simulink model "PMSM_My_PI_Simscapes"  (R2017b)
settings: Solver=VariableStepAuto  StartTime=0.0  StopTime=0.2  FixedStep=0.000001  MaxStep=1e-4  RelTol=1e-3
undefined symbols (not defined in the file or in its folder): sigbuilder_block
libraries: fl_lib x46, nesl_utility x28, elec_lib x13, powerlib x2, simulink x1
settings Model: Creator=Linyc  LastModifiedBy=Crazyyiwen
settings DebuggingCC: UnconnectedLineMsg=none

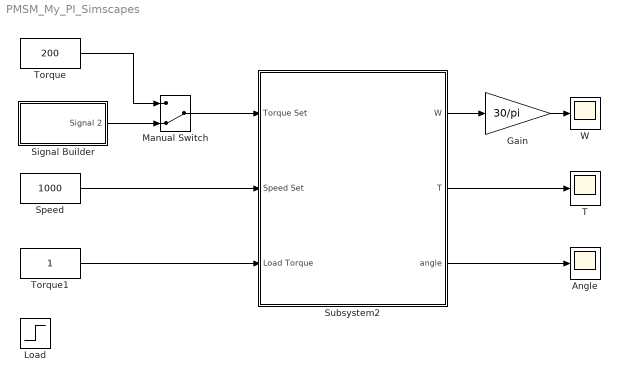
== system PMSM_My_PI_Simscapes ==
  Angle : Scope
  Gain : Gain  Gain=30/pi
  Load : Step  Time=0.02  After=0  SampleTime=0
  Manual Switch : ManualSwitch  CurrentSetting=0
  Signal Builder : Subsystem  Tag=STV Subsys  LoadFcn=sigbuilder_block('load');  StartFcn=sigbuilder_block('start');  StopFcn=sigbuilder_block('stop');  ClipboardFcn=sigbuilder_block('clipboard');  mask(Sigbuilder block){tuvar=[0:10]}
      mask help: Simulink:masks:SigbuilderBlock_MD
      mask init:
      | if ~strcmp(get_param(bdroot(gcbh),'SimulationStatus'),'stopped') tuvar = sigbuilder_block('maskInit'); end
      settings: CopyFcn=sigbuilder_block('copy');  DeleteFcn=sigbuilder_block('delete');  ModelCloseFcn=sigbuilder_block('modelClose');  PreSaveFcn=sigbuilder_block('preSave');  PauseFcn=sigbuilder_block('pause');  ContinueFcn=sigbuilder_block('continue');  NameChangeFcn=sigbuilder_block('namechange');  OpenFcn=sigbuilder_block('open',[424.5 166.5 847.5 399.75 ]);  CloseFcn=sigbuilder_block('close');
      mask Display: plot(0, 0, 100, 100,[2, 2, 32, 32, 2], [68, 8, 8, 68, 68],[32, 2], [38, 38], [32, 19, 2],[53, 60, 44], [32, 17, 17, 2],[16, 16, 31, 31]);txt = getActiveGroup(gcbh);text(2, 100, txt,'verticalAlignment', 'top');
  Speed : Constant  Value=1000
  Subsystem2 : Subsystem
  T : Scope
  Torque : Constant  Value=200
  Torque1 : Constant
  W : Scope
  wires:
  Speed/1 -> Subsystem2/2(Speed Set)
  Subsystem2/1(W) -> Gain/1
  Subsystem2/2(T) -> T/1
  Subsystem2/3(angle) -> Angle/1
  Gain/1 -> W/1
  Torque/1 -> Manual Switch/1
  Manual Switch/1 -> Subsystem2/1(Torque Set)
  Signal Builder/1(Signal 2) -> Manual Switch/2
  Torque1/1 -> Subsystem2/3(Load Torque)

== system PMSM_My_PI_Simscapes/Signal Builder ==
  Demux : Demux  Tag=STV Demux  Outputs=1
  FromWs : FromWorkspace  Tag=STV FromWs  VariableName=tuvar  SampleTime=0
      SigBuilderData=|
      | common.afterFinalStr = 'Extrapolate'
      | common.sampleTime = 0
      | dataSet.timeRange = [0 2]
      | dataSet.name = 'Group 1'
      | sbobj.Groups.Name = 'Group 1'
      | sbobj.Groups.Signals.Name = 'Signal 2'
      | sbobj.Groups.Signals.XData = [0 1 1 2]
      | sbobj.Groups.Signals.YData = [200 200 0 0]
      | sbobj.Groups.TimeRange = [0 2]
  Signal 2 : Outport  Tag=STV Outport
  wires:
  FromWs/1 -> Demux/1
  Demux/1 -> Signal 2/1

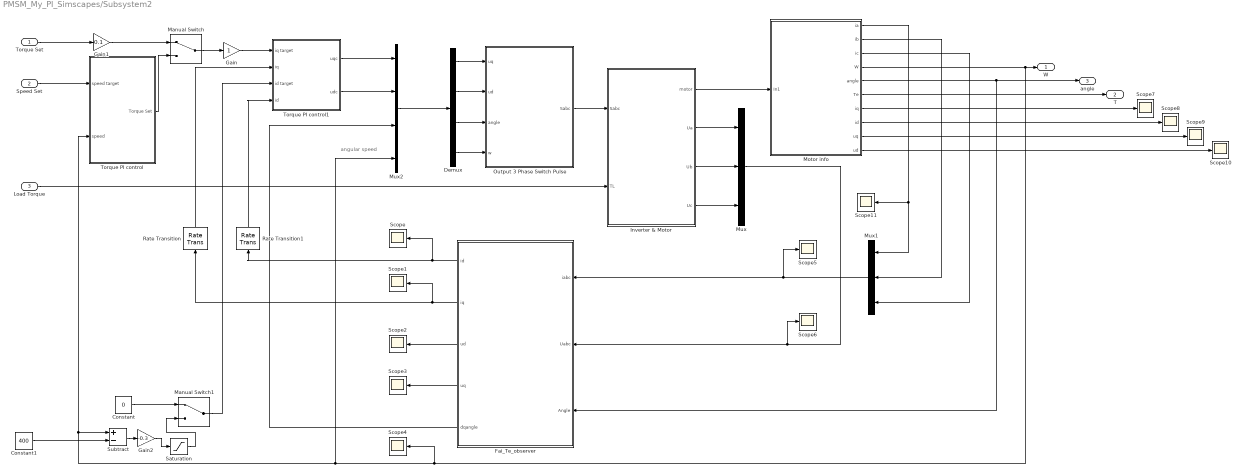
== system PMSM_My_PI_Simscapes/Subsystem2 ==
  note: angular speed
  Torque Set : Inport
  Speed Set : Inport  Port=2
  Load Torque : Inport  Port=3
  Constant : Constant  Value=0
  Constant1 : Constant  Value=400
  Demux : Demux
  Fai_Te_observer : Subsystem
  Gain : Gain
  Gain1 : Gain  Gain=0.1
  Gain2 : Gain  Gain=-0.3
  Inverter & Motor : Subsystem
  Manual Switch : ManualSwitch
  Manual Switch1 : ManualSwitch
  Motor info : Subsystem
  Mux : Mux  Inputs=3
  Mux1 : Mux  Inputs=3
  Mux2 : Mux
  Output 3 Phase Switch Pulse : Subsystem
  Rate Transition : RateTransition  OutPortSampleTime=0.0002
  Rate Transition1 : RateTransition  OutPortSampleTime=0.0002
  Saturation : Saturate  UpperLimit=0  LowerLimit=-150
  Scope{,1..11} (12 alike) : Scope
  Subtract : Sum  Inputs=+-
  Torque PI control : Subsystem
  Torque PI control1 : Subsystem
  W : Outport
  T : Outport  Port=2
  angle : Outport  Port=3
  wires:
  Motor info/4(W) -> Scope4/1, Mux2/4, Subtract/1, Torque PI control/2(speed), W/1
  Load Torque/1 -> Inverter & Motor/2(TL)
  Inverter & Motor/2(Ua) -> Mux/1
  Inverter & Motor/4(Uc) -> Mux/3
  Inverter & Motor/3(Ub) -> Mux/2
  Motor info/6(Te) -> T/1
  Inverter & Motor/1(motor) -> Motor info/1(In1)
  Motor info/5(angle) -> Fai_Te_observer/3(Angle), angle/1
  Motor info/1(ia) -> Scope11/1, Mux1/1
  Motor info/2(ib) -> Mux1/2
  Motor info/3(ic) -> Mux1/3
  Output 3 Phase Switch Pulse/1(Sabc) -> Inverter & Motor/1(Sabc)
  Mux1/1 -> Fai_Te_observer/1(iabc), Scope5/1
  Mux/1 -> Fai_Te_observer/2(Uabc), Scope6/1
  Mux2/1 -> Demux/1
  Motor info/7(iq) -> Scope7/1
  Motor info/8(id) -> Scope8/1
  Motor info/9(uq) -> Scope9/1
  Motor info/10(ud) -> Scope10/1
  Fai_Te_observer/1(id) -> Rate Transition1/1, Scope/1
  Fai_Te_observer/2(iq) -> Rate Transition/1, Scope1/1
  Fai_Te_observer/3(ud) -> Scope2/1
  Fai_Te_observer/4(uq) -> Scope3/1
  Speed Set/1 -> Torque PI control/1(speed target)
  Torque Set/1 -> Gain1/1
  Torque PI control/1(Torque Set) -> Manual Switch/2
  Fai_Te_observer/5(dqangle) -> Mux2/3
  Manual Switch/1 -> Gain/1
  Gain/1 -> Torque PI control1/1(iq target)
  Demux/1 -> Output 3 Phase Switch Pulse/1(uq)
  Demux/2 -> Output 3 Phase Switch Pulse/2(ud)
  Demux/3 -> Output 3 Phase Switch Pulse/3(angle)
  Torque PI control1/1(uqc) -> Mux2/1
  Rate Transition/1 -> Torque PI control1/2(iq)
  Demux/4 -> Output 3 Phase Switch Pulse/4(w)
  Gain1/1 -> Manual Switch/1
  Torque PI control1/2(udc) -> Mux2/2
  Rate Transition1/1 -> Torque PI control1/4(id)
  Constant/1 -> Manual Switch1/1
  Manual Switch1/1 -> Torque PI control1/3(id target)
  Constant1/1 -> Subtract/2
  Subtract/1 -> Gain2/1
  Gain2/1 -> Saturation/1
  Saturation/1 -> Manual Switch1/2

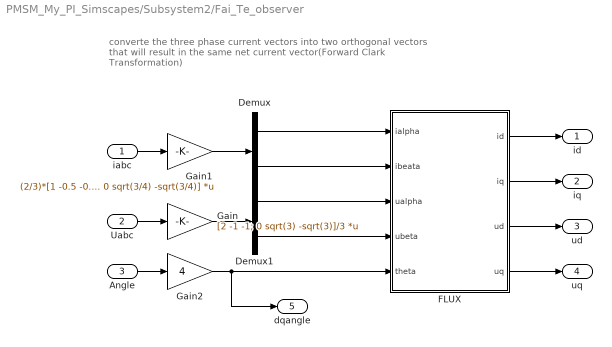
== system PMSM_My_PI_Simscapes/Subsystem2/Fai_Te_observer ==
  note: converte the three phase current vectors into
      | two orthogonal vectors that will result in the
      | same net current vector(Forward Clark Transformation)
  iabc : Inport
  Uabc : Inport  Port=2
  Angle : Inport  Port=3
  Demux : Demux  Outputs=2
  Demux1 : Demux  Outputs=2
  FLUX : Subsystem
  Gain : Gain  Gain=[2 -1 -1; 0 sqrt(3) -sqrt(3)]/3  Multiplication=Matrix(K*u)
  Gain1 : Gain  Gain=(2/3)*[1 -0.5 -0.5; 0 sqrt(3/4) -sqrt(3/4)]  Multiplication=Matrix(K*u)
  Gain2 : Gain  Gain=4
  id : Outport
  iq : Outport  Port=2
  ud : Outport  Port=3
  uq : Outport  Port=4
  dqangle : Outport  Port=5
  wires:
  Demux/1 -> FLUX/1(ialpha)
  Gain/1 -> Demux1/1
  iabc/1 -> Gain1/1
  Demux/2 -> FLUX/2(ibeata)
  Demux1/2 -> FLUX/4(ubeta)
  Demux1/1 -> FLUX/3(ualpha)
  Uabc/1 -> Gain/1
  Gain1/1 -> Demux/1
  Angle/1 -> Gain2/1
  Gain2/1 -> dqangle/1, FLUX/5(theta)
  FLUX/1(id) -> id/1
  FLUX/2(iq) -> iq/1
  FLUX/3(ud) -> ud/1
  FLUX/4(uq) -> uq/1

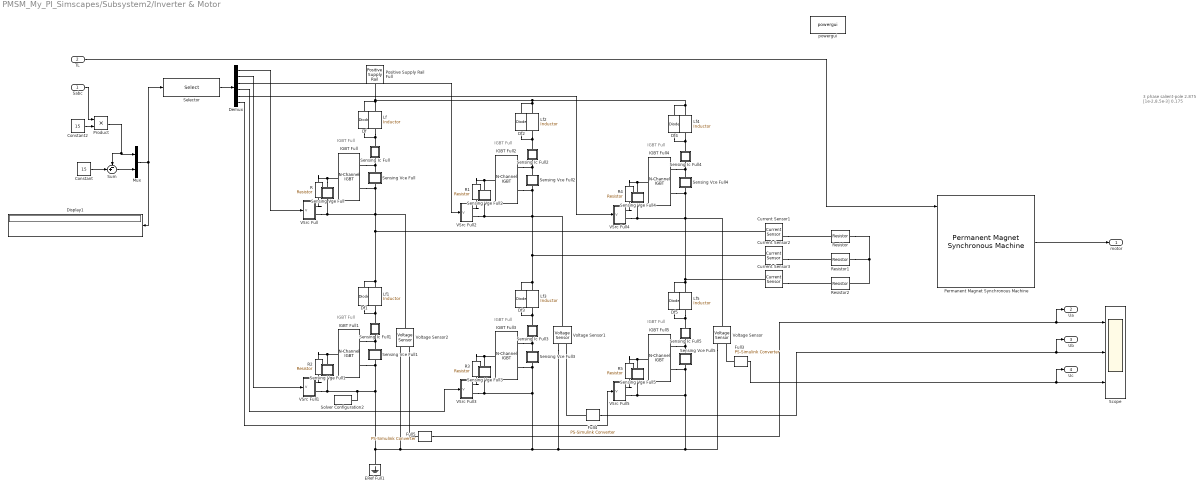
== system PMSM_My_PI_Simscapes/Subsystem2/Inverter & Motor ==
  note: 3 phase
      | salient-pole
      |
      | 2.875
      | [1e-2,8.5e-3]
      | 0.175
  note: IGBT
      | Full
  note: IGBT
      | Full
  note: IGBT
      | Full
  note: IGBT
      | Full
  note: IGBT
      | Full
  note: IGBT
      | Full
  Sabc : Inport
  TL : Inport  Port=2
  Constant : Constant  Value=15
  Constant2 : Constant  Value=15
  Current Sensor1 : fl_lib/Electrical/Electrical Sensors/Current Sensor
      settings: SourceProductName=Foundation Library
  Current Sensor2 : fl_lib/Electrical/Electrical Sensors/Current Sensor
      settings: SourceProductName=Foundation Library
  Current Sensor3 : fl_lib/Electrical/Electrical Sensors/Current Sensor
      settings: SourceProductName=Foundation Library
  Demux : Demux  Outputs=6
  Df{,1..5} (6 alike) : elec_lib/Semiconductor Devices/Diode  ModelType=3  Vf=0.6 V  Ron=0.01 Ohm  Goff=1e-5 S  Rz=0.3 Ohm  Vz=50 V  C_PWL=50 pF  prmExp=1  I12="[ 3  30 ] A"  V12=[ 0.8 1.1 ] V  I1=0.0137 A  V1=0.6 V  IS=1e-12 A  ec=1  RS=0.01 Ohm  Tmeas=25 degC  BV=Inf V  C_param=1  CJ0=1 nF  VJ=1 V  Mgrad=0.5  Vvec=[ 0.1 10 100 ] V  Cvec=[ 3.5 1 0.4 ] pF  FC=0.5  Q_param=2  Irrm=-100 A  iF=200 A  didt=-1000 A/us  trr=115 ns  TT=50 ns  tau=100 ns  T_param=1  IS_T2=1.25e-7 A  I1_T2=0.245 A  V1_T2=0.5 V  Tmeas2=125 degC  EG_param=1  EG=1.11 eV  XTI_param=1  XTI=3  dBVdT=0 V/K  Tdevice=25 degC  i_capacitor_specify=off  i_capacitor_priority=High  i_capacitor=0 A  i_capacitor_nominal_specify=off  i_capacitor_nominal_unit=A  i_capacitor_nominal_value=1  v_capacitor_specify=off  v_capacitor_priority=None  v_capacitor=0 V  v_capacitor_nominal_specify=off  v_capacitor_nominal_unit=V  v_capacitor_nominal_value=1  Rth=[ 0 10 ] K/W  thermal_mass_parameterization=1  thermal_mass=[ 0 1 ] J/K  thermal_time_constant=[ 0 10 ] s  thermal_mass_initial_temperatures=[ 25 25 ] degC
      settings: SourceProductName=Simscape Electronics  SourceProductBaseCode=SN
  Display1 : Display
  ERef Full1 : fl_lib/Electrical/Electrical Elements/Electrical Reference
      settings: SourceProductName=Foundation Library
  Full3 : nesl_utility/PS-Simulink Converter  PhysicalDomain=network_engine_domain  SubClassName=ps_output  LeftPortType=input  RightPortType=output  PseudoPeriodic=off  Frequencies=[]  Unit=1  AffineConversion=off
  Full4 : nesl_utility/PS-Simulink Converter  PhysicalDomain=network_engine_domain  SubClassName=ps_output  LeftPortType=input  RightPortType=output  PseudoPeriodic=off  Frequencies=[]  Unit=1  AffineConversion=off
  Full5 : nesl_utility/PS-Simulink Converter  PhysicalDomain=network_engine_domain  SubClassName=ps_output  LeftPortType=input  RightPortType=output  PseudoPeriodic=off  Frequencies=[]  Unit=1  AffineConversion=off
  IGBT Full{,1..5} (6 alike) : elec_lib/Semiconductor Devices/N-Channel IGBT  model_type=1  Ices=2 mA  Vces=600 V  Vth=6 V  Vce_sat=2.6 V  Ice_sat=300 A  Vge_sat=15 V  ec=3  Tmeas=25 degC  Vge_vec=[ -2 6 7 8 10 12 15 20 ] V  Vce_vec=[0, 1.1, 1.3, 1.45, 1.75, 2.25, 2.7] V  T_vec=[25, 125] degC  Ic_mat=[ -1.015e-5 1.35e-8 4.7135e-4 5.092e-4 5.105e-4 5.117500000000001e-4 5.1299e-4 5.1423e-4 5.1548e-4 5.1672e-4; -9.986899999999999e-6 1.35e-8 4.7135e-4 5.092e-4 5.105e-4 5.117500000000001e-4 5.1299e-4 5.1423e-4 5.1548e-4 5.1672e-4; -9.955e-6 1.35e-8 0.0065225 3.3324 48.154 93.661 105.52 105.72 105.93 106.14; -9.955e-6 1.35e-8 0.0065235 3.5783 70.264 166.33 252.4 317.67 353.38 357.39; -9.955e-6 1.35e-8 0.006524 3.7206 89.17100000000001 228.09 371.63 511.02 642.6900000000001 764.04; -9.9549e-6 1.35e-8 0.0065242 3.7716 97.79300000000001 256.21 424.27 592.92 759.2 921.52; -9.9549e-6 1.35e-8 0.0065243 3.8067 104.52 278.11 464.6 654.37 844.5700000000001 1.0339e+3; -9.9549e-6 1.35e-8 0.0065244 3.8324 109.92 295.67 496.54 702.28 909.96 1.1183e+3 ] A  Ic_mat_3D=zeros(8, 10, 2) A  C_param=1  C_GE=23.7 nF  C_GC=2.7 nF  C_CE=0 nF  C_ies=26.4 nF  C_res=2.7 nF  C_oes=0 nF  C_GE_vec=[ 25 31 26.5 24.9 25 24.9 24.6 24.7 24.8 ] nF  C_GC_vec=[ 55 9 5.5 3.1 2.5 2.1 1.9 1.8 1.7 ] nF  C_CE_vec=[ 5 11 6.5 4.9 3.5 2.7 2.1 1.7 1.4 ] nF  C_ies_vec=[ 80 40 32 28 27.5 27 26.5 26.5 26.5 ] nF  C_res_vec=[ 55 9 5.5 3.1 2.5 2.1 1.9 1.8 1.7 ] nF  C_oes_vec=[ 55 20 12 8 6 4.8 4 3.5 3.1 ] nF  C_Vce_vec=[ 0 1 2 5 10 15 20 25 30 ] V  charge_linearity_param=2  C_OX=50 nF  V_C_OX=-4 V  TF=150 us  VAF=200 V  RC=0.001 Ohm  RE=0.001 Ohm  RG=0.001 Ohm  BF=1  T_param=1  Ices_T2=100 mA  EG=1.11 eV  Vce_sat_T2=3 V  Tmeas2=125 degC  XTI=3  BEX=-1.5  RG_alpha=0 1/K  Tdevice=25 degC  Tdevice_3D=25 degC  Rth=[0, 10] K/W  thermal_mass_parameterization=1  thermal_mass=[0, 1] J/K  thermal_time_constant=[0, 10] s  thermal_mass_initial_temperatures=[298.15, 298.15] K  Ic_vec1=[0, 10, 50, 100, 200, 400, 600] A  Vce_vec1=[0, 1.1, 1.3, 1.45, 1.75, 2.25, 2.7] V  Rmiller=0.12 Ohm  Goff=1e-5 1/Ohm  t_on=0.09 us  t_rise=0.7 us  t_off=0.2 us  t_fall=0.4 us  v_meas=300 V  Tj_vec1=[298.15, 398.15] K  Vce_mat1=[0, 1.1, 1.3, 1.45, 1.75, 2.25, 2.7; 0, 1.0, 1.15, 1.35, 1.7, 2.35, 3.0] V  E_turn_on_mat1=[0, 0.2, 1, 2, 4, 8, 15; 0, 0.3, 1.3, 2.5, 5, 11, 18] * 1e-3 J  E_turn_off_mat1=[0, 0.3, 1.5, 3, 6, 15, 25; 0, 0.7, 3.3, 6.5, 13, 25, 35] * 1e-3 J
      settings: SourceProductName=Simscape Electronics  SourceProductBaseCode=SN
  Lf{,1..5} (6 alike) : fl_lib/Electrical/Electrical Elements/Inductor  l=0.5e-5 H  r=1e-4 Ohm  g=1e-6 1/Ohm  i_specify=off  i_priority=High  i=0 A  i_nominal_specify=off  i_nominal_unit=A  i_nominal_value=1  v_specify=off  v_priority=High  v=0 V  v_nominal_specify=off  v_nominal_unit=V  v_nominal_value=1  i_L_specify=on  i_L_priority=High  i_L=0 A  i_L_nominal_specify=off  i_L_nominal_unit=A  i_L_nominal_value=1
      settings: SourceProductName=Foundation Library
  Mux : Mux  Inputs=2
  Permanent Magnet Synchronous Machine : powerlib/Machines/Permanent Magnet Synchronous Machine  NbPhases=3  FluxDistribution=Sinusoidal  RotorType=Salient-pole  MechanicalLoad=Torque Tm  PresetModel=No  ShowDetailedParameters=on  MeasurementBus=off  Resistance=2.875  Inductance=8.5e-3  dqInductances=[1e-2,8.5e-3]  La=0.000395  MachineConstant=Flux linkage established by magnets (V.s)  Flux=0.175  VoltageCst=126.966  TorqueCst=1.05  Flat=120  Mechanical=[0.0027 0.175 4 0]  PolePairs=2  InitialConditions=[0,0, 0,0]  InitialConditions5ph=[0 0 0 0 0 0]  TsPowergui=0  TsBlock=-1  RefAngle=Aligned with phase A axis (original Park)
      settings: SourceProductName=Simscape Power Systems
  Positive Supply Rail Full : elec_lib/Sources/Positive Supply Rail  v0=380 V
      settings: SourceProductName=Simscape Electronics  SourceProductBaseCode=SN
  Product : Product
  R{,1..5} (6 alike) : fl_lib/Electrical/Electrical Elements/Resistor  R=4.7 Ohm  i_specify=off  i_priority=High  i=0 A  i_nominal_specify=off  i_nominal_unit=A  i_nominal_value=1  v_specify=off  v_priority=High  v=0 V  v_nominal_specify=off  v_nominal_unit=V  v_nominal_value=1
      settings: SourceProductName=Foundation Library
  Resistor : fl_lib/Electrical/Electrical Elements/Resistor  R=5 Ohm  i_specify=off  i_priority=None  i=0 A  i_nominal_specify=off  i_nominal_unit=A  i_nominal_value=1  v_specify=off  v_priority=None  v=0 V  v_nominal_specify=off  v_nominal_unit=V  v_nominal_value=1
  Resistor1 : fl_lib/Electrical/Electrical Elements/Resistor  R=5 Ohm  i_specify=off  i_priority=None  i=0 A  i_nominal_specify=off  i_nominal_unit=A  i_nominal_value=1  v_specify=off  v_priority=None  v=0 V  v_nominal_specify=off  v_nominal_unit=V  v_nominal_value=1
  Resistor2 : fl_lib/Electrical/Electrical Elements/Resistor  R=5 Ohm  i_specify=off  i_priority=None  i=0 A  i_nominal_specify=off  i_nominal_unit=A  i_nominal_value=1  v_specify=off  v_priority=None  v=0 V  v_nominal_specify=off  v_nominal_unit=V  v_nominal_value=1
  Scope : Scope  NumInputPorts=3
  Selector : Selector  InputPortWidth=6  IndexOptions=Index vector (dialog)  Indices=[1 4 2 5 3 6]  OutputSizes=1
  Sensing Ic Full : Subsystem
      mask Display: disp('Ic')
  Sensing Ic Full1 : Subsystem
      mask Display: disp('Ic')
  Sensing Ic Full2 : Subsystem
      mask Display: disp('Ic')
  Sensing Ic Full3 : Subsystem
      mask Display: disp('Ic')
  Sensing Ic Full4 : Subsystem
      mask Display: disp('Ic')
  Sensing Ic Full5 : Subsystem
      mask Display: disp('Ic')
  Sensing Vce Full : Subsystem
      mask Display: disp('Vce')
  Sensing Vce Full1 : Subsystem
      mask Display: disp('Vce')
  Sensing Vce Full2 : Subsystem
      mask Display: disp('Vce')
  Sensing Vce Full3 : Subsystem
      mask Display: disp('Vce')
  Sensing Vce Full4 : Subsystem
      mask Display: disp('Vce')
  Sensing Vce Full5 : Subsystem
      mask Display: disp('Vce')
  Sensing Vge Full : Subsystem
      mask Display: disp('Vge')
  Sensing Vge Full1 : Subsystem
      mask Display: disp('Vge')
  Sensing Vge Full2 : Subsystem
      mask Display: disp('Vge')
  Sensing Vge Full3 : Subsystem
      mask Display: disp('Vge')
  Sensing Vge Full4 : Subsystem
      mask Display: disp('Vge')
  Sensing Vge Full5 : Subsystem
      mask Display: disp('Vge')
  Solver Configuration2 : nesl_utility/Solver Configuration  PhysicalDomain=network_engine_domain  SubClassName=solver  LeftPortType=input  RightPortType=generic  Accelerate=off  Tones=[]  Harmonics=[]  SimulateNoise=off  Profile=off  UseLocalSampling=off  EnableSwitchedLinearOptims=on  FrequencyDomain=off  UseCCode=off  RelTol=0.001  AbsTol=1e-06  MinStep=1e-09  ToWorkspace=off  RevertToSquareIcSolve=off  NumHomotopyIterations=100  PhasorMode=off  PhasorModeNumHarmonics=1  DoDC=off  ResidualTolerance=1e-6  UseLocalSolver=off  LocalSolverChoice=NE_BACKWARD_EULER_ADVANCER  LocalSolverSampleTime=1e-6  DoFixedCost=off  MaxNonlinIter=3  MaxModeIter=2  LinearAlgebra=Sparse  DelaysMemoryBudget=1024  AutomaticFiltering=on  FilteringTimeConstant=0.001
  Sum : Sum  Inputs=-+|
  VSrc Full : Subsystem
      settings: CopyFcn=set_param(gcb,'LinkStatus','none')
  VSrc Full1 : Subsystem
      settings: CopyFcn=set_param(gcb,'LinkStatus','none')
  VSrc Full2 : Subsystem
      settings: CopyFcn=set_param(gcb,'LinkStatus','none')
  VSrc Full3 : Subsystem
      settings: CopyFcn=set_param(gcb,'LinkStatus','none')
  VSrc Full4 : Subsystem
      settings: CopyFcn=set_param(gcb,'LinkStatus','none')
  VSrc Full5 : Subsystem
      settings: CopyFcn=set_param(gcb,'LinkStatus','none')
  Voltage Sensor : fl_lib/Electrical/Electrical Sensors/Voltage Sensor
      settings: SourceProductName=Foundation Library
  Voltage Sensor1 : fl_lib/Electrical/Electrical Sensors/Voltage Sensor
      settings: SourceProductName=Foundation Library
  Voltage Sensor2 : fl_lib/Electrical/Electrical Sensors/Voltage Sensor
      settings: SourceProductName=Foundation Library
  powergui : powerlib/powergui  Priority=1  SimulationMode=Continuous  SampleTime=0.000001  frequency=60  Iterations=50  frequencyindice=0  Pbase=100e6  ErrMax=1e-4  UnitsV=kV  UnitsW=MW  buscounter=0  FunctionMessages=off  echomessages=off  EnableUseOfTLC=off  CurrentSourceSwitches=off  DisableSnubberDevices=off  DisableRonSwitches=off  DisableVfSwitches=off  DisplayEquations=off  SolverType=Tustin/Backward Euler (TBE)  Interpol=off  ExternalGateDelay=off  methode=off  Ts=100  x0status=blocks  SPID=on  SwTol=0  HookPort=off  RestoreLinks=warning  ResistiveCurrentMeasurement=off  Frange=[0:2:500]  Ylog=off  Xlog=on  ShowGrid=off  save=off  variable=ZData  structure=0  ZoomFFT=off  StartTime=0.0  cycles=1  DisplayStyle=1  fundamental=60  FreqAxis=off  MaxFrequency=1000  frequencyindicesteady=1  RmsSteady=1  display=off
  motor : Outport
  Ua : Outport  Port=2
  Ub : Outport  Port=3
  Uc : Outport  Port=4
  wires:
  Constant/1 -> Sum/2
  Sum/1 -> Mux/2
  Mux/1 -> Display1/1, Selector/1
  Full5/1 -> Ua/1, Scope/1
  Full4/1 -> Ub/1, Scope/2
  Full3/1 -> Uc/1, Scope/3
  Permanent Magnet Synchronous Machine/1 -> motor/1
  Selector/1 -> Demux/1
  Constant2/1 -> Product/2
  Sabc/1 -> Product/1
  Product/1 -> Sum/1, Mux/1
  Demux/1 -> VSrc Full/1(V)
  Demux/2 -> VSrc Full1/1(V)
  Demux/3 -> VSrc Full2/1(V)
  Demux/4 -> VSrc Full3/1(V)
  Demux/5 -> VSrc Full4/1(V)
  Demux/6 -> VSrc Full5/1(V)
  TL/1 -> Permanent Magnet Synchronous Machine/1
  connections:
  Sensing Vge Full/LConn1 -- R/RConn1 -- IGBT Full/LConn1
  Df3/RConn1 -- Current Sensor2/LConn1 -- Sensing Vge Full2/RConn1 -- VSrc Full2/RConn2 -- Voltage Sensor1/LConn1 -- Sensing Vce Full2/RConn1 -- IGBT Full2/RConn2 -- Lf3/LConn1
  Sensing Vce Full5/LConn1 -- IGBT Full5/RConn1 -- Sensing Ic Full5/RConn1
  IGBT Full2/LConn1 -- Sensing Vge Full2/LConn1 -- R1/RConn1
  Lf4/RConn1 -- Sensing Ic Full4/LConn1 -- Df4/LConn1
  Lf2/RConn1 -- Sensing Ic Full2/LConn1 -- Df2/LConn1
  Lf1/RConn1 -- Sensing Ic Full1/LConn1 -- Df1/LConn1
  R3/RConn1 -- IGBT Full3/LConn1 -- Sensing Vge Full3/LConn1
  Df5/RConn1 -- Current Sensor3/LConn1 -- Sensing Vge Full4/RConn1 -- VSrc Full4/RConn2 -- Voltage Sensor/LConn1 -- Sensing Vce Full4/RConn1 -- IGBT Full4/RConn2 -- Lf5/LConn1
  IGBT Full3/RConn2 -- Voltage Sensor/RConn2 -- Sensing Vge Full5/RConn1 -- VSrc Full5/RConn2 -- Sensing Vce Full5/RConn1 -- IGBT Full5/RConn2 -- Voltage Sensor1/RConn2 -- Voltage Sensor2/RConn2 -- Sensing Vce Full1/RConn1 -- IGBT Full1/RConn2 -- Solver Configuration2/RConn1 -- VSrc Full1/RConn2 -- Sensing Vge Full1/RConn1 -- ERef Full1/LConn1 -- VSrc Full3/RConn2 -- Sensing Vge Full3/RConn1 -- Sensing Vce Full3/RConn1
  R5/RConn1 -- IGBT Full5/LConn1 -- Sensing Vge Full5/LConn1
  IGBT Full1/LConn1 -- Sensing Vge Full1/LConn1 -- R2/RConn1
  IGBT Full4/LConn1 -- Sensing Vge Full4/LConn1 -- R4/RConn1
  Df3/LConn1 -- Lf3/RConn1 -- Sensing Ic Full3/LConn1
  Sensing Ic Full/RConn1 -- Sensing Vce Full/LConn1 -- IGBT Full/RConn1
  Sensing Vce Full3/LConn1 -- IGBT Full3/RConn1 -- Sensing Ic Full3/RConn1
  IGBT Full4/RConn1 -- Sensing Ic Full4/RConn1 -- Sensing Vce Full4/LConn1
  Lf/LConn1 -- Df/RConn1 -- Lf4/LConn1 -- Df4/RConn1 -- Df2/RConn1 -- Lf2/LConn1 -- Positive Supply Rail Full/RConn1
  IGBT Full1/RConn1 -- Sensing Ic Full1/RConn1 -- Sensing Vce Full1/LConn1
  Df5/LConn1 -- Lf5/RConn1 -- Sensing Ic Full5/LConn1
  Sensing Ic Full/LConn1 -- Df/LConn1 -- Lf/RConn1
  IGBT Full2/RConn1 -- Sensing Ic Full2/RConn1 -- Sensing Vce Full2/LConn1
  VSrc Full/RConn1 -- R/LConn1
  VSrc Full2/RConn1 -- R1/LConn1
  VSrc Full4/RConn1 -- R4/LConn1
  VSrc Full5/RConn1 -- R5/LConn1
  VSrc Full3/RConn1 -- R3/LConn1
  VSrc Full1/RConn1 -- R2/LConn1
  Full3/LConn1 -- Voltage Sensor/RConn1
  Full4/LConn1 -- Voltage Sensor1/RConn1
  Full5/LConn1 -- Voltage Sensor2/RConn1
  Df1/RConn1 -- Current Sensor1/LConn1 -- VSrc Full/RConn2 -- Sensing Vge Full/RConn1 -- Voltage Sensor2/LConn1 -- Sensing Vce Full/RConn1 -- IGBT Full/RConn2 -- Lf1/LConn1
  Resistor/RConn1 -- Resistor1/RConn1 -- Resistor2/RConn1
  Current Sensor2/RConn2 -- Resistor1/LConn1
  Current Sensor1/RConn2 -- Resistor/LConn1
  Current Sensor3/RConn2 -- Resistor2/LConn1

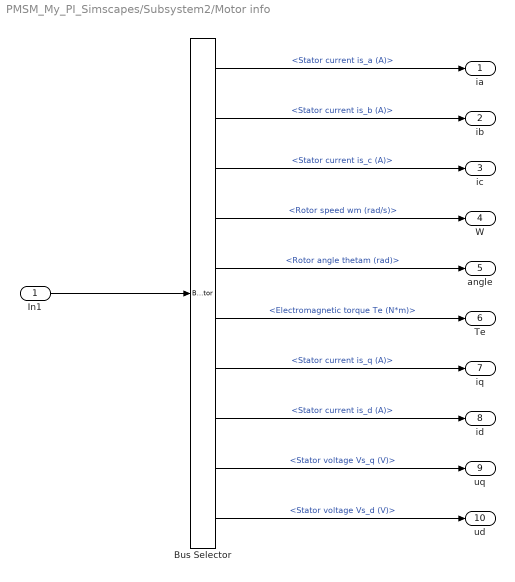
== system PMSM_My_PI_Simscapes/Subsystem2/Motor info ==
  In1 : Inport
  Bus Selector : BusSelector  OutputSignals=Stator current is_a (A),Stator current is_b (A),Stator current is_c (A),Rotor speed wm (rad/s),Rotor angle thetam (rad),Electromagnetic torque Te (N*m),Stator current is_q (A),Stator current is_d (A),Stator voltage Vs_q (V),Stator voltage Vs_d (V)
  ia : Outport
  ib : Outport  Port=2
  ic : Outport  Port=3
  W : Outport  Port=4
  angle : Outport  Port=5
  Te : Outport  Port=6
  iq : Outport  Port=7
  id : Outport  Port=8
  uq : Outport  Port=9
  ud : Outport  Port=10
  wires:
  In1/1 -> Bus Selector/1
  Bus Selector/2 -> ib/1  "<Stator current is_b (A)>"
  Bus Selector/3 -> ic/1  "<Stator current is_c (A)>"
  Bus Selector/6 -> Te/1  "<Electromagnetic torque Te (N*m)>"
  Bus Selector/1 -> ia/1  "<Stator current is_a (A)>"
  Bus Selector/5 -> angle/1  "<Rotor angle thetam (rad)>"
  Bus Selector/4 -> W/1  "<Rotor speed wm (rad/s)>"
  Bus Selector/7 -> iq/1  "<Stator current is_q (A)>"
  Bus Selector/8 -> id/1  "<Stator current is_d (A)>"
  Bus Selector/9 -> uq/1  "<Stator voltage Vs_q (V)>"
  Bus Selector/10 -> ud/1  "<Stator voltage Vs_d (V)>"

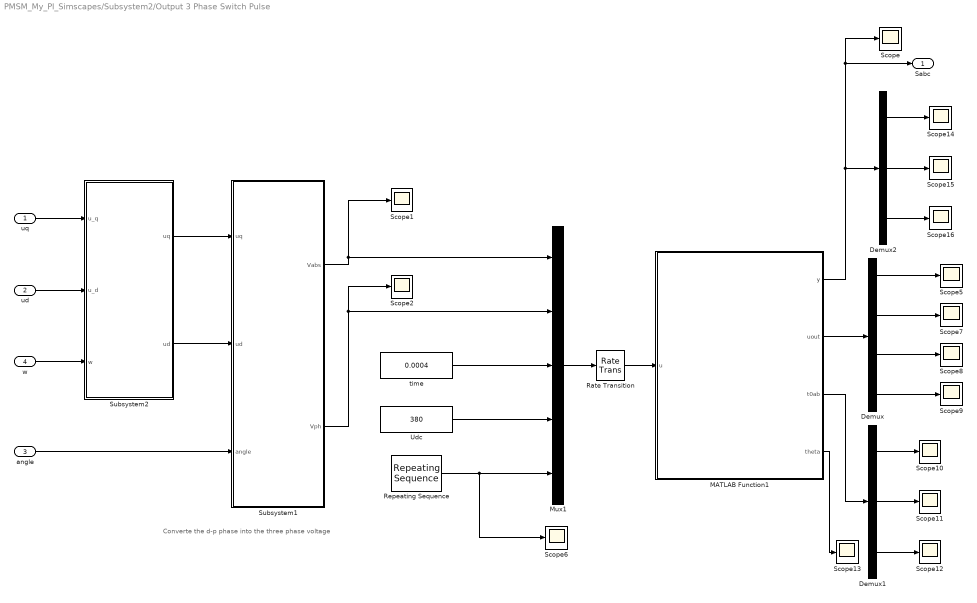
== system PMSM_My_PI_Simscapes/Subsystem2/Output 3 Phase Switch Pulse ==
  note: Converte the d-p phase into the three phase voltage
  uq : Inport
  ud : Inport  Port=2
  angle : Inport  Port=3
  w : Inport  Port=4
  Demux : Demux
  Demux1 : Demux  Outputs=3
  Demux2 : Demux  Outputs=3
  MATLAB Function1 : MATLAB Function  TreatAsAtomicUnit=on
  Mux1 : Mux  Inputs=5
  Rate Transition : RateTransition  OutPortSampleTime=0.000001
  Repeating Sequence : simulink/Sources/Repeating Sequence  rep_seq_t=[0 0.0002 0.0004]  rep_seq_y=[0 380 0]
  Scope{,1..2,5..16} (15 alike) : Scope
  Subsystem1 : Subsystem
  Subsystem2 : Subsystem
  Udc : Constant  Value=380
  time : Constant  Value=0.0004
  Sabc : Outport
  wires:
  time/1 -> Mux1/3
  Repeating Sequence/1 -> Scope6/1, Mux1/5
  Udc/1 -> Mux1/4
  MATLAB Function1/1(y) -> Demux2/1, Scope/1, Sabc/1
  Subsystem1/1(Vabs) -> Mux1/1, Scope1/1
  Subsystem1/2(Vph) -> Mux1/2, Scope2/1
  Mux1/1 -> Rate Transition/1
  MATLAB Function1/2(uout) -> Demux/1
  Demux/4 -> Scope9/1
  Demux/2 -> Scope7/1
  Demux/3 -> Scope8/1
  Demux/1 -> Scope5/1
  MATLAB Function1/3(t0ab) -> Demux1/1
  Demux1/1 -> Scope10/1
  Demux1/3 -> Scope12/1
  Demux1/2 -> Scope11/1
  MATLAB Function1/4(theta) -> Scope13/1
  Demux2/2 -> Scope15/1
  Demux2/3 -> Scope16/1
  Demux2/1 -> Scope14/1
  Rate Transition/1 -> MATLAB Function1/1(u)
  uq/1 -> Subsystem2/1(u_q)
  ud/1 -> Subsystem2/2(u_d)
  Subsystem2/1(uq) -> Subsystem1/1(uq)
  Subsystem2/2(ud) -> Subsystem1/2(ud)
  angle/1 -> Subsystem1/3(angle)
  w/1 -> Subsystem2/3(w)

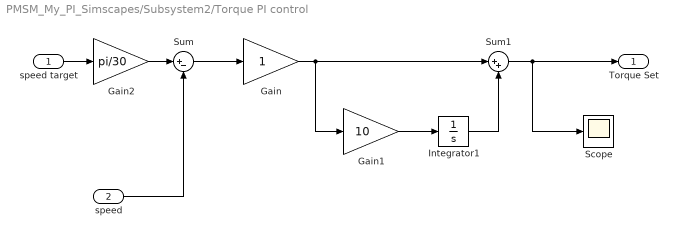
== system PMSM_My_PI_Simscapes/Subsystem2/Torque PI control ==
  speed target : Inport
  speed : Inport  Port=2
  Gain : Gain
  Gain1 : Gain  Gain=10
  Gain2 : Gain  Gain=pi/30
  Integrator1 : Integrator
  Scope : Scope
  Sum : Sum  Inputs=|+-
  Sum1 : Sum  Inputs=|++
  Torque Set : Outport
  wires:
  speed target/1 -> Gain2/1
  Sum/1 -> Gain/1
  speed/1 -> Sum/2
  Gain2/1 -> Sum/1
  Gain/1 -> Gain1/1, Sum1/1
  Integrator1/1 -> Sum1/2
  Sum1/1 -> Scope/1, Torque Set/1
  Gain1/1 -> Integrator1/1

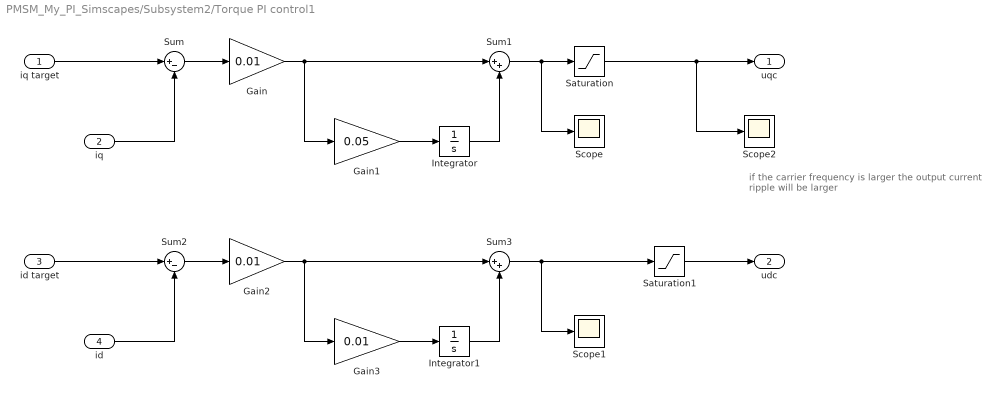
== system PMSM_My_PI_Simscapes/Subsystem2/Torque PI control1 ==
  note: if the carrier frequency is larger the
      | output current ripple will be larger
  iq target : Inport
  iq : Inport  Port=2
  id target : Inport  Port=3
  id : Inport  Port=4
  Gain : Gain  Gain=0.01
  Gain1 : Gain  Gain=0.05
  Gain2 : Gain  Gain=0.01
  Gain3 : Gain  Gain=0.01
  Integrator : Integrator
  Integrator1 : Integrator
  Saturation : Saturate  UpperLimit=1  LowerLimit=-1
  Saturation1 : Saturate  UpperLimit=1  LowerLimit=-1
  Scope : Scope
  Scope1 : Scope
  Scope2 : Scope
  Sum : Sum  Inputs=|+-
  Sum1 : Sum  Inputs=|++
  Sum2 : Sum  Inputs=|+-
  Sum3 : Sum  Inputs=|++
  uqc : Outport
  udc : Outport  Port=2
  wires:
  Gain1/1 -> Integrator/1
  Integrator/1 -> Sum1/2
  Gain/1 -> Gain1/1, Sum1/1
  iq/1 -> Sum/2
  Sum/1 -> Gain/1
  id target/1 -> Sum2/1
  Sum2/1 -> Gain2/1
  id/1 -> Sum2/2
  Gain2/1 -> Sum3/1, Gain3/1
  Sum3/1 -> Saturation1/1, Scope1/1
  Integrator1/1 -> Sum3/2
  Gain3/1 -> Integrator1/1
  Saturation1/1 -> udc/1
  iq target/1 -> Sum/1
  Sum1/1 -> Saturation/1, Scope/1
  Saturation/1 -> Scope2/1, uqc/1

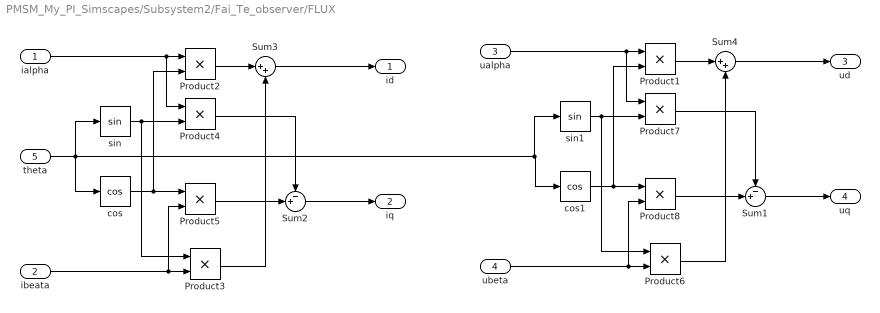
== system PMSM_My_PI_Simscapes/Subsystem2/Fai_Te_observer/FLUX ==
  ialpha : Inport
  ibeata : Inport  Port=2
  ualpha : Inport  Port=3
  ubeta : Inport  Port=4
  theta : Inport  Port=5
  Product{1..8} (8 alike) : Product
  Sum1 : Sum  Inputs=-+|
  Sum2 : Sum  Inputs=-+|
  Sum3 : Sum  Inputs=|++
  Sum4 : Sum  Inputs=|++
  cos : Trigonometry  Operator=cos
  cos1 : Trigonometry  Operator=cos
  sin : Trigonometry
  sin1 : Trigonometry
  id : Outport
  iq : Outport  Port=2
  ud : Outport  Port=3
  uq : Outport  Port=4
  wires:
  ialpha/1 -> Product4/1, Product2/1
  cos/1 -> Product5/1, Product2/2
  ibeata/1 -> Product5/2, Product3/2
  sin/1 -> Product4/2, Product3/1
  Product2/1 -> Sum3/1
  Product3/1 -> Sum3/2
  Product4/1 -> Sum2/1
  Product5/1 -> Sum2/2
  Sum3/1 -> id/1
  Sum2/1 -> iq/1
  Sum1/1 -> uq/1
  Sum4/1 -> ud/1
  Product8/1 -> Sum1/2
  Product7/1 -> Sum1/1
  Product6/1 -> Sum4/2
  Product1/1 -> Sum4/1
  sin1/1 -> Product6/1, Product7/2
  ubeta/1 -> Product6/2, Product8/2
  cos1/1 -> Product1/2, Product8/1
  ualpha/1 -> Product1/1, Product7/1
  theta/1 -> sin1/1, cos1/1, sin/1, cos/1

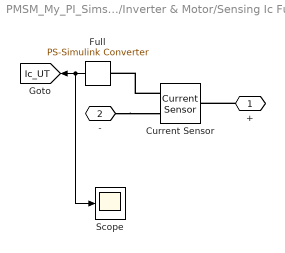
== system PMSM_My_PI_Simscapes/Subsystem2/Inverter & Motor/Sensing Ic Full ==
  Current Sensor : fl_lib/Electrical/Electrical Sensors/Current Sensor
      settings: SourceProductName=Foundation Library
  Full : nesl_utility/PS-Simulink Converter  PhysicalDomain=network_engine_domain  SubClassName=ps_output  LeftPortType=input  RightPortType=output  PseudoPeriodic=off  Frequencies=[]  Unit=1  AffineConversion=off
  Scope : Scope
  + : PMIOPort  Port=1  Side=Left
  - : PMIOPort  Port=2  Side=Right
  tag scope: Ic_UT=global
  wires:
  Full/1 -> Scope/1, [Ic_UT]
  connections:
  Current Sensor/RConn1 -- Full/LConn1
  -/RConn1 -- Current Sensor/RConn2
  +/RConn1 -- Current Sensor/LConn1

== system PMSM_My_PI_Simscapes/Subsystem2/Inverter & Motor/Sensing Ic Full1 ==
  Current Sensor : fl_lib/Electrical/Electrical Sensors/Current Sensor
      settings: SourceProductName=Foundation Library
  Full : nesl_utility/PS-Simulink Converter  PhysicalDomain=network_engine_domain  SubClassName=ps_output  LeftPortType=input  RightPortType=output  PseudoPeriodic=off  Frequencies=[]  Unit=1  AffineConversion=off
  Scope : Scope
  + : PMIOPort  Port=1  Side=Left
  - : PMIOPort  Port=2  Side=Right
  tag scope: Ic_UB=global
  wires:
  Full/1 -> Scope/1, [Ic_UB]
  connections:
  Current Sensor/RConn1 -- Full/LConn1
  -/RConn1 -- Current Sensor/RConn2
  +/RConn1 -- Current Sensor/LConn1

== system PMSM_My_PI_Simscapes/Subsystem2/Inverter & Motor/Sensing Ic Full2 ==
  Current Sensor : fl_lib/Electrical/Electrical Sensors/Current Sensor
      settings: SourceProductName=Foundation Library
  Full : nesl_utility/PS-Simulink Converter  PhysicalDomain=network_engine_domain  SubClassName=ps_output  LeftPortType=input  RightPortType=output  PseudoPeriodic=off  Frequencies=[]  Unit=1  AffineConversion=off
  Scope : Scope
  + : PMIOPort  Port=1  Side=Left
  - : PMIOPort  Port=2  Side=Right
  tag scope: Ic_VT=global
  wires:
  Full/1 -> Scope/1, [Ic_VT]
  connections:
  Current Sensor/RConn1 -- Full/LConn1
  -/RConn1 -- Current Sensor/RConn2
  +/RConn1 -- Current Sensor/LConn1

== system PMSM_My_PI_Simscapes/Subsystem2/Inverter & Motor/Sensing Ic Full3 ==
  Current Sensor : fl_lib/Electrical/Electrical Sensors/Current Sensor
      settings: SourceProductName=Foundation Library
  Full : nesl_utility/PS-Simulink Converter  PhysicalDomain=network_engine_domain  SubClassName=ps_output  LeftPortType=input  RightPortType=output  PseudoPeriodic=off  Frequencies=[]  Unit=1  AffineConversion=off
  Scope : Scope
  + : PMIOPort  Port=1  Side=Left
  - : PMIOPort  Port=2  Side=Right
  tag scope: Ic_VB=global
  wires:
  Full/1 -> Scope/1, [Ic_VB]
  connections:
  Current Sensor/RConn1 -- Full/LConn1
  -/RConn1 -- Current Sensor/RConn2
  +/RConn1 -- Current Sensor/LConn1

== system PMSM_My_PI_Simscapes/Subsystem2/Inverter & Motor/Sensing Ic Full4 ==
  Current Sensor : fl_lib/Electrical/Electrical Sensors/Current Sensor
      settings: SourceProductName=Foundation Library
  Full : nesl_utility/PS-Simulink Converter  PhysicalDomain=network_engine_domain  SubClassName=ps_output  LeftPortType=input  RightPortType=output  PseudoPeriodic=off  Frequencies=[]  Unit=1  AffineConversion=off
  Scope : Scope
  + : PMIOPort  Port=1  Side=Left
  - : PMIOPort  Port=2  Side=Right
  tag scope: Ic_WT=global
  wires:
  Full/1 -> Scope/1, [Ic_WT]
  connections:
  Current Sensor/RConn1 -- Full/LConn1
  -/RConn1 -- Current Sensor/RConn2
  +/RConn1 -- Current Sensor/LConn1

== system PMSM_My_PI_Simscapes/Subsystem2/Inverter & Motor/Sensing Ic Full5 ==
  Current Sensor : fl_lib/Electrical/Electrical Sensors/Current Sensor
      settings: SourceProductName=Foundation Library
  Full : nesl_utility/PS-Simulink Converter  PhysicalDomain=network_engine_domain  SubClassName=ps_output  LeftPortType=input  RightPortType=output  PseudoPeriodic=off  Frequencies=[]  Unit=1  AffineConversion=off
  Scope : Scope
  + : PMIOPort  Port=1  Side=Left
  - : PMIOPort  Port=2  Side=Right
  tag scope: Ic_WB=global
  wires:
  Full/1 -> Scope/1, [Ic_WB]
  connections:
  Current Sensor/RConn1 -- Full/LConn1
  -/RConn1 -- Current Sensor/RConn2
  +/RConn1 -- Current Sensor/LConn1

== system PMSM_My_PI_Simscapes/Subsystem2/Inverter & Motor/Sensing Vce Full ==
  Full : nesl_utility/PS-Simulink Converter  PhysicalDomain=network_engine_domain  SubClassName=ps_output  LeftPortType=input  RightPortType=output  PseudoPeriodic=off  Frequencies=[]  Unit=V  AffineConversion=off
  Scope : Scope
  Voltage Sensor : fl_lib/Electrical/Electrical Sensors/Voltage Sensor
      settings: SourceProductName=Foundation Library
  + : PMIOPort  Port=1  Side=Left
  - : PMIOPort  Port=2  Side=Right
  tag scope: Vce_UT=global
  wires:
  Full/1 -> Scope/1, [Vce_UT]
  connections:
  Voltage Sensor/RConn1 -- Full/LConn1
  -/RConn1 -- Voltage Sensor/RConn2
  Voltage Sensor/LConn1 -- +/RConn1

== system PMSM_My_PI_Simscapes/Subsystem2/Inverter & Motor/Sensing Vce Full1 ==
  Full : nesl_utility/PS-Simulink Converter  PhysicalDomain=network_engine_domain  SubClassName=ps_output  LeftPortType=input  RightPortType=output  PseudoPeriodic=off  Frequencies=[]  Unit=V  AffineConversion=off
  Scope : Scope
  Voltage Sensor : fl_lib/Electrical/Electrical Sensors/Voltage Sensor
      settings: SourceProductName=Foundation Library
  + : PMIOPort  Port=1  Side=Left
  - : PMIOPort  Port=2  Side=Right
  tag scope: Vce_UB=global
  wires:
  Full/1 -> Scope/1, [Vce_UB]
  connections:
  Voltage Sensor/RConn1 -- Full/LConn1
  -/RConn1 -- Voltage Sensor/RConn2
  Voltage Sensor/LConn1 -- +/RConn1

== system PMSM_My_PI_Simscapes/Subsystem2/Inverter & Motor/Sensing Vce Full2 ==
  Full : nesl_utility/PS-Simulink Converter  PhysicalDomain=network_engine_domain  SubClassName=ps_output  LeftPortType=input  RightPortType=output  PseudoPeriodic=off  Frequencies=[]  Unit=V  AffineConversion=off
  Scope : Scope
  Voltage Sensor : fl_lib/Electrical/Electrical Sensors/Voltage Sensor
      settings: SourceProductName=Foundation Library
  + : PMIOPort  Port=1  Side=Left
  - : PMIOPort  Port=2  Side=Right
  tag scope: Vce_VT=global
  wires:
  Full/1 -> Scope/1, [Vce_VT]
  connections:
  Voltage Sensor/RConn1 -- Full/LConn1
  -/RConn1 -- Voltage Sensor/RConn2
  Voltage Sensor/LConn1 -- +/RConn1

== system PMSM_My_PI_Simscapes/Subsystem2/Inverter & Motor/Sensing Vce Full3 ==
  Full : nesl_utility/PS-Simulink Converter  PhysicalDomain=network_engine_domain  SubClassName=ps_output  LeftPortType=input  RightPortType=output  PseudoPeriodic=off  Frequencies=[]  Unit=V  AffineConversion=off
  Scope : Scope
  Voltage Sensor : fl_lib/Electrical/Electrical Sensors/Voltage Sensor
      settings: SourceProductName=Foundation Library
  + : PMIOPort  Port=1  Side=Left
  - : PMIOPort  Port=2  Side=Right
  tag scope: Vce_VB=global
  wires:
  Full/1 -> Scope/1, [Vce_VB]
  connections:
  Voltage Sensor/RConn1 -- Full/LConn1
  -/RConn1 -- Voltage Sensor/RConn2
  Voltage Sensor/LConn1 -- +/RConn1

== system PMSM_My_PI_Simscapes/Subsystem2/Inverter & Motor/Sensing Vce Full4 ==
  Full : nesl_utility/PS-Simulink Converter  PhysicalDomain=network_engine_domain  SubClassName=ps_output  LeftPortType=input  RightPortType=output  PseudoPeriodic=off  Frequencies=[]  Unit=V  AffineConversion=off
  Scope : Scope
  Voltage Sensor : fl_lib/Electrical/Electrical Sensors/Voltage Sensor
      settings: SourceProductName=Foundation Library
  + : PMIOPort  Port=1  Side=Left
  - : PMIOPort  Port=2  Side=Right
  tag scope: Vce_WT=global
  wires:
  Full/1 -> Scope/1, [Vce_WT]
  connections:
  Voltage Sensor/RConn1 -- Full/LConn1
  -/RConn1 -- Voltage Sensor/RConn2
  Voltage Sensor/LConn1 -- +/RConn1

== system PMSM_My_PI_Simscapes/Subsystem2/Inverter & Motor/Sensing Vce Full5 ==
  Full : nesl_utility/PS-Simulink Converter  PhysicalDomain=network_engine_domain  SubClassName=ps_output  LeftPortType=input  RightPortType=output  PseudoPeriodic=off  Frequencies=[]  Unit=V  AffineConversion=off
  Scope : Scope
  Voltage Sensor : fl_lib/Electrical/Electrical Sensors/Voltage Sensor
      settings: SourceProductName=Foundation Library
  + : PMIOPort  Port=1  Side=Left
  - : PMIOPort  Port=2  Side=Right
  tag scope: Vce_WB=global
  wires:
  Full/1 -> Scope/1, [Vce_WB]
  connections:
  Voltage Sensor/RConn1 -- Full/LConn1
  -/RConn1 -- Voltage Sensor/RConn2
  Voltage Sensor/LConn1 -- +/RConn1

== system PMSM_My_PI_Simscapes/Subsystem2/Inverter & Motor/Sensing Vge Full ==
  Full : nesl_utility/PS-Simulink Converter  PhysicalDomain=network_engine_domain  SubClassName=ps_output  LeftPortType=input  RightPortType=output  PseudoPeriodic=off  Frequencies=[]  Unit=V  AffineConversion=off
  Voltage Sensor : fl_lib/Electrical/Electrical Sensors/Voltage Sensor
      settings: SourceProductName=Foundation Library
  + : PMIOPort  Port=1  Side=Left
  - : PMIOPort  Port=2  Side=Right
  tag scope: Vge_UT=global
  wires:
  Full/1 -> [Vge_UT]
  connections:
  Voltage Sensor/RConn1 -- Full/LConn1
  -/RConn1 -- Voltage Sensor/RConn2
  Voltage Sensor/LConn1 -- +/RConn1

== system PMSM_My_PI_Simscapes/Subsystem2/Inverter & Motor/Sensing Vge Full1 ==
  Full : nesl_utility/PS-Simulink Converter  PhysicalDomain=network_engine_domain  SubClassName=ps_output  LeftPortType=input  RightPortType=output  PseudoPeriodic=off  Frequencies=[]  Unit=V  AffineConversion=off
  Voltage Sensor : fl_lib/Electrical/Electrical Sensors/Voltage Sensor
      settings: SourceProductName=Foundation Library
  + : PMIOPort  Port=1  Side=Left
  - : PMIOPort  Port=2  Side=Right
  tag scope: Vge_UB=global
  wires:
  Full/1 -> [Vge_UB]
  connections:
  Voltage Sensor/RConn1 -- Full/LConn1
  -/RConn1 -- Voltage Sensor/RConn2
  Voltage Sensor/LConn1 -- +/RConn1

== system PMSM_My_PI_Simscapes/Subsystem2/Inverter & Motor/Sensing Vge Full2 ==
  Full : nesl_utility/PS-Simulink Converter  PhysicalDomain=network_engine_domain  SubClassName=ps_output  LeftPortType=input  RightPortType=output  PseudoPeriodic=off  Frequencies=[]  Unit=V  AffineConversion=off
  Voltage Sensor : fl_lib/Electrical/Electrical Sensors/Voltage Sensor
      settings: SourceProductName=Foundation Library
  + : PMIOPort  Port=1  Side=Left
  - : PMIOPort  Port=2  Side=Right
  tag scope: Vge_VT=global
  wires:
  Full/1 -> [Vge_VT]
  connections:
  Voltage Sensor/RConn1 -- Full/LConn1
  -/RConn1 -- Voltage Sensor/RConn2
  Voltage Sensor/LConn1 -- +/RConn1

== system PMSM_My_PI_Simscapes/Subsystem2/Inverter & Motor/Sensing Vge Full3 ==
  Full : nesl_utility/PS-Simulink Converter  PhysicalDomain=network_engine_domain  SubClassName=ps_output  LeftPortType=input  RightPortType=output  PseudoPeriodic=off  Frequencies=[]  Unit=V  AffineConversion=off
  Voltage Sensor : fl_lib/Electrical/Electrical Sensors/Voltage Sensor
      settings: SourceProductName=Foundation Library
  + : PMIOPort  Port=1  Side=Left
  - : PMIOPort  Port=2  Side=Right
  tag scope: Vge_VB=global
  wires:
  Full/1 -> [Vge_VB]
  connections:
  Voltage Sensor/RConn1 -- Full/LConn1
  -/RConn1 -- Voltage Sensor/RConn2
  Voltage Sensor/LConn1 -- +/RConn1

== system PMSM_My_PI_Simscapes/Subsystem2/Inverter & Motor/Sensing Vge Full4 ==
  Full : nesl_utility/PS-Simulink Converter  PhysicalDomain=network_engine_domain  SubClassName=ps_output  LeftPortType=input  RightPortType=output  PseudoPeriodic=off  Frequencies=[]  Unit=V  AffineConversion=off
  Voltage Sensor : fl_lib/Electrical/Electrical Sensors/Voltage Sensor
      settings: SourceProductName=Foundation Library
  + : PMIOPort  Port=1  Side=Left
  - : PMIOPort  Port=2  Side=Right
  tag scope: Vge_WT=global
  wires:
  Full/1 -> [Vge_WT]
  connections:
  Voltage Sensor/RConn1 -- Full/LConn1
  -/RConn1 -- Voltage Sensor/RConn2
  Voltage Sensor/LConn1 -- +/RConn1

== system PMSM_My_PI_Simscapes/Subsystem2/Inverter & Motor/Sensing Vge Full5 ==
  Full : nesl_utility/PS-Simulink Converter  PhysicalDomain=network_engine_domain  SubClassName=ps_output  LeftPortType=input  RightPortType=output  PseudoPeriodic=off  Frequencies=[]  Unit=V  AffineConversion=off
  Voltage Sensor : fl_lib/Electrical/Electrical Sensors/Voltage Sensor
      settings: SourceProductName=Foundation Library
  + : PMIOPort  Port=1  Side=Left
  - : PMIOPort  Port=2  Side=Right
  tag scope: Vge_WB=global
  wires:
  Full/1 -> [Vge_WB]
  connections:
  Voltage Sensor/RConn1 -- Full/LConn1
  -/RConn1 -- Voltage Sensor/RConn2
  Voltage Sensor/LConn1 -- +/RConn1

== system PMSM_My_PI_Simscapes/Subsystem2/Inverter & Motor/VSrc Full ==
  V : Inport
  Controlled Voltage Source : fl_lib/Electrical/Electrical Sources/Controlled Voltage Source
      settings: SourceProductName=Foundation Library
  Simulink-PS Converter : nesl_utility/Simulink-PS Converter  PhysicalDomain=network_engine_domain  SubClassName=ps_input  LeftPortType=input  RightPortType=output  PseudoPeriodic=off  Frequencies=[]  NoiseDistribution=none  NoiseParameters=[]  Unit=V  AffineConversion=off  FilteringAndDerivatives=zero  SimscapeFilterOrder=1  InputFilterTimeConstant=.001  UdotUserProvided=0
  + : PMIOPort  Port=1  Side=Right
  - : PMIOPort  Port=2  Side=Right
  wires:
  V/1 -> Simulink-PS Converter/1
  connections:
  Controlled Voltage Source/RConn1 -- Simulink-PS Converter/RConn1
  -/RConn1 -- Controlled Voltage Source/RConn2
  +/RConn1 -- Controlled Voltage Source/LConn1

== system PMSM_My_PI_Simscapes/Subsystem2/Inverter & Motor/VSrc Full1 ==
  V : Inport
  Controlled Voltage Source : fl_lib/Electrical/Electrical Sources/Controlled Voltage Source
      settings: SourceProductName=Foundation Library
  Simulink-PS Converter : nesl_utility/Simulink-PS Converter  PhysicalDomain=network_engine_domain  SubClassName=ps_input  LeftPortType=input  RightPortType=output  PseudoPeriodic=off  Frequencies=[]  NoiseDistribution=none  NoiseParameters=[]  Unit=V  AffineConversion=off  FilteringAndDerivatives=zero  SimscapeFilterOrder=1  InputFilterTimeConstant=.001  UdotUserProvided=0
  + : PMIOPort  Port=1  Side=Right
  - : PMIOPort  Port=2  Side=Right
  wires:
  V/1 -> Simulink-PS Converter/1
  connections:
  Controlled Voltage Source/RConn1 -- Simulink-PS Converter/RConn1
  -/RConn1 -- Controlled Voltage Source/RConn2
  +/RConn1 -- Controlled Voltage Source/LConn1

== system PMSM_My_PI_Simscapes/Subsystem2/Inverter & Motor/VSrc Full2 ==
  V : Inport
  Controlled Voltage Source : fl_lib/Electrical/Electrical Sources/Controlled Voltage Source
      settings: SourceProductName=Foundation Library
  Simulink-PS Converter : nesl_utility/Simulink-PS Converter  PhysicalDomain=network_engine_domain  SubClassName=ps_input  LeftPortType=input  RightPortType=output  PseudoPeriodic=off  Frequencies=[]  NoiseDistribution=none  NoiseParameters=[]  Unit=V  AffineConversion=off  FilteringAndDerivatives=zero  SimscapeFilterOrder=1  InputFilterTimeConstant=.001  UdotUserProvided=0
  + : PMIOPort  Port=1  Side=Right
  - : PMIOPort  Port=2  Side=Right
  wires:
  V/1 -> Simulink-PS Converter/1
  connections:
  Controlled Voltage Source/RConn1 -- Simulink-PS Converter/RConn1
  -/RConn1 -- Controlled Voltage Source/RConn2
  +/RConn1 -- Controlled Voltage Source/LConn1

== system PMSM_My_PI_Simscapes/Subsystem2/Inverter & Motor/VSrc Full3 ==
  V : Inport
  Controlled Voltage Source : fl_lib/Electrical/Electrical Sources/Controlled Voltage Source
      settings: SourceProductName=Foundation Library
  Simulink-PS Converter : nesl_utility/Simulink-PS Converter  PhysicalDomain=network_engine_domain  SubClassName=ps_input  LeftPortType=input  RightPortType=output  PseudoPeriodic=off  Frequencies=[]  NoiseDistribution=none  NoiseParameters=[]  Unit=V  AffineConversion=off  FilteringAndDerivatives=zero  SimscapeFilterOrder=1  InputFilterTimeConstant=.001  UdotUserProvided=0
  + : PMIOPort  Port=1  Side=Right
  - : PMIOPort  Port=2  Side=Right
  wires:
  V/1 -> Simulink-PS Converter/1
  connections:
  Controlled Voltage Source/RConn1 -- Simulink-PS Converter/RConn1
  -/RConn1 -- Controlled Voltage Source/RConn2
  +/RConn1 -- Controlled Voltage Source/LConn1

== system PMSM_My_PI_Simscapes/Subsystem2/Inverter & Motor/VSrc Full4 ==
  V : Inport
  Controlled Voltage Source : fl_lib/Electrical/Electrical Sources/Controlled Voltage Source
      settings: SourceProductName=Foundation Library
  Simulink-PS Converter : nesl_utility/Simulink-PS Converter  PhysicalDomain=network_engine_domain  SubClassName=ps_input  LeftPortType=input  RightPortType=output  PseudoPeriodic=off  Frequencies=[]  NoiseDistribution=none  NoiseParameters=[]  Unit=V  AffineConversion=off  FilteringAndDerivatives=zero  SimscapeFilterOrder=1  InputFilterTimeConstant=.001  UdotUserProvided=0
  + : PMIOPort  Port=1  Side=Right
  - : PMIOPort  Port=2  Side=Right
  wires:
  V/1 -> Simulink-PS Converter/1
  connections:
  Controlled Voltage Source/RConn1 -- Simulink-PS Converter/RConn1
  -/RConn1 -- Controlled Voltage Source/RConn2
  +/RConn1 -- Controlled Voltage Source/LConn1

== system PMSM_My_PI_Simscapes/Subsystem2/Inverter & Motor/VSrc Full5 ==
  V : Inport
  Controlled Voltage Source : fl_lib/Electrical/Electrical Sources/Controlled Voltage Source
      settings: SourceProductName=Foundation Library
  Simulink-PS Converter : nesl_utility/Simulink-PS Converter  PhysicalDomain=network_engine_domain  SubClassName=ps_input  LeftPortType=input  RightPortType=output  PseudoPeriodic=off  Frequencies=[]  NoiseDistribution=none  NoiseParameters=[]  Unit=V  AffineConversion=off  FilteringAndDerivatives=zero  SimscapeFilterOrder=1  InputFilterTimeConstant=.001  UdotUserProvided=0
  + : PMIOPort  Port=1  Side=Right
  - : PMIOPort  Port=2  Side=Right
  wires:
  V/1 -> Simulink-PS Converter/1
  connections:
  Controlled Voltage Source/RConn1 -- Simulink-PS Converter/RConn1
  -/RConn1 -- Controlled Voltage Source/RConn2
  +/RConn1 -- Controlled Voltage Source/LConn1

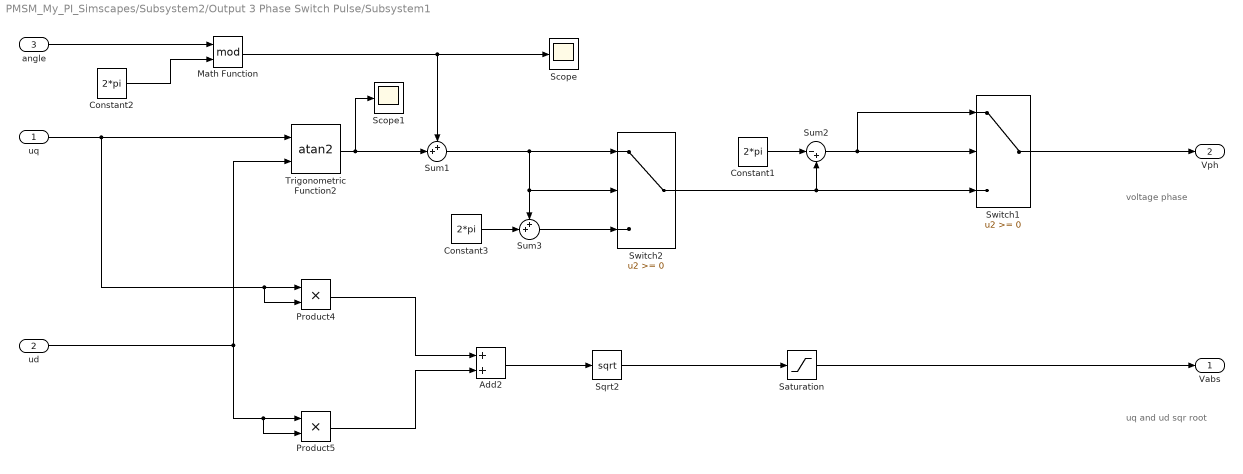
== system PMSM_My_PI_Simscapes/Subsystem2/Output 3 Phase Switch Pulse/Subsystem1 ==
  note: voltage phase
  note: uq and ud sqr root
  uq : Inport
  ud : Inport  Port=2
  angle : Inport  Port=3
  Add2 : Sum
  Constant1 : Constant  Value=2*pi
  Constant2 : Constant  Value=2*pi
  Constant3 : Constant  Value=2*pi
  Math Function : Math  Operator=mod  SaturateOnIntegerOverflow=on
  Product4 : Product
  Product5 : Product
  Saturation : Saturate  UpperLimit=380  LowerLimit=0
  Scope : Scope
  Scope1 : Scope
  Sqrt2 : Sqrt  SaturateOnIntegerOverflow=on
  Sum1 : Sum  Inputs=++|
  Sum2 : Sum  Inputs=|-+
  Sum3 : Sum  Inputs=++|
  Switch1 : Switch
  Switch2 : Switch
  Trigonometric Function2 : Trigonometry  Operator=atan2
  Vabs : Outport
  Vph : Outport  Port=2
  wires:
  Product5/1 -> Add2/2
  ud/1 -> Trigonometric Function2/2, Product5/2, Product5/1
  Sqrt2/1 -> Saturation/1
  Product4/1 -> Add2/1
  Add2/1 -> Sqrt2/1
  uq/1 -> Trigonometric Function2/1, Product4/2, Product4/1
  Sum3/1 -> Switch2/3
  Sum1/1 -> Sum3/1, Switch2/2, Switch2/1
  Constant3/1 -> Sum3/2
  Trigonometric Function2/1 -> Scope1/1, Sum1/2
  Sum2/1 -> Switch1/2, Switch1/1
  Constant1/1 -> Sum2/1
  Switch2/1 -> Switch1/3, Sum2/2
  Switch1/1 -> Vph/1
  angle/1 -> Math Function/1
  Constant2/1 -> Math Function/2
  Math Function/1 -> Scope/1, Sum1/1
  Saturation/1 -> Vabs/1

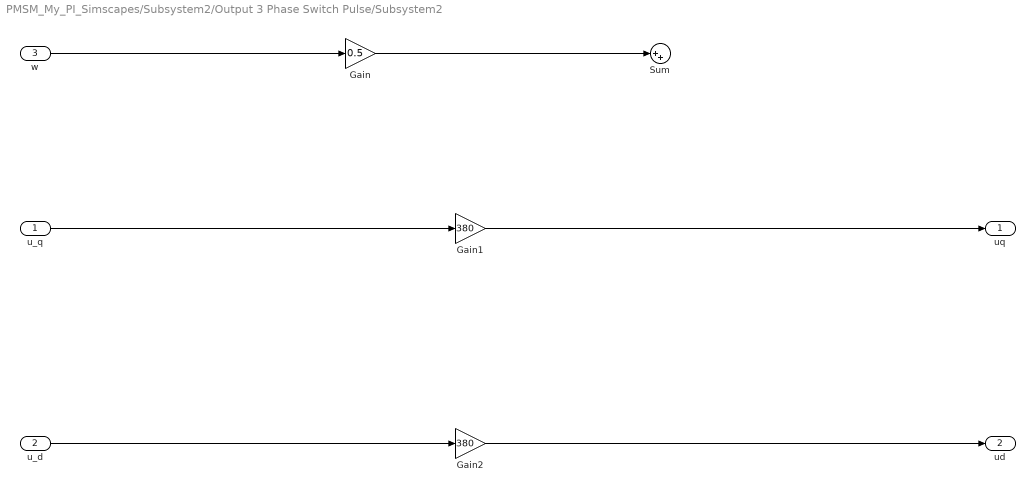
== system PMSM_My_PI_Simscapes/Subsystem2/Output 3 Phase Switch Pulse/Subsystem2 ==
  u_q : Inport
  u_d : Inport  Port=2
  w : Inport  Port=3
  Gain : Gain  Gain=0.5
  Gain1 : Gain  Gain=380
  Gain2 : Gain  Gain=380
  Sum : Sum  Inputs=|++
  uq : Outport
  ud : Outport  Port=2
  wires:
  u_d/1 -> Gain2/1
  w/1 -> Gain/1
  Gain/1 -> Sum/1
  u_q/1 -> Gain1/1
  Gain1/1 -> uq/1
  Gain2/1 -> ud/1

== matlab function PMSM_My_PI_Simscapes/Subsystem2/Output 3 Phase Switch Pulse/MATLAB Function1 ==
  data: u input size=5; y output; uout output; t0ab output; theta output
function [y, uout, t0ab,theta] = svpwm005(u)
Vabs=u(1);
ph=u(2);
tp=u(3);
Udc=u(4);
du=pi/3;

% define 8 vectors
u0=[0 0 0];
u1=[0 0 1];
u2=[0 1 0];
u3=[0 1 1];
u4=[1 0 0];
u5=[1 0 1];
u6=[1 1 0];
u7=[1 1 1];

% determine which sector ph belongs to
if ph>0 && ph<=du
    theta=ph;
    h=1;
    ua=u4;
    ub=u6;
elseif ph>du && ph<=2*du
    theta=2*du-ph;
    h=2;
    ua=u2;
    ub=u6;
elseif ph>2*du && ph<=3*du
    theta=ph-2*du;
    h=3;
    ua=u2;
    ub=u3;
elseif ph>3*du && ph<=4*du
    theta=4*du-ph;
    h=4;
    ua=u1;
    ub=u3;
elseif ph>4*du && ph<=5*du
    theta=ph-4*du;
    h=5;
    ua=u1;
    ub=u5;
else
    theta=6*du-ph;
    h=6;
    ua=u4;
    ub=u5;
end

% calculate ta,tb,tc
ta=1.5*(cos(theta)-1/sqrt(3)*sin(theta))*Vabs*tp/Udc;
tb=sqrt(3)*Vabs*sin(theta)*tp/Udc;
t0=tp-ta-tb;
if t0<0
    ta=ta/(ta+tb)*tp;
    tb=tp-ta;
    t0=0;
end
% transfor the time into the voltage
usw1=Udc*t0/tp/2;
usw2=Udc*ta/tp+usw1;
usw3=Udc*tb/tp+usw2;
%判断并输出
if u(5)>=0 && u(5)<usw1
    y=u0;
elseif u(5)>=usw1 && u(5)<usw2
    y=ua;
elseif u(5)>=usw2 && u(5)<usw3
    y=ub;
else
    y=u7;
end
uout=[usw1 usw2 usw3 u(5)];
t0ab=[t0 ta tb];
